simulink model "Project_adp_posmeas2_ver2"  (Simulink 7.3)
settings: Solver=ode45  StartTime=0.0  StopTime=25  RelTol=1e-3
libraries: dspmtrx3 x6, simulink x4
settings Model: Creator=GILL  LastModifiedBy=GILL

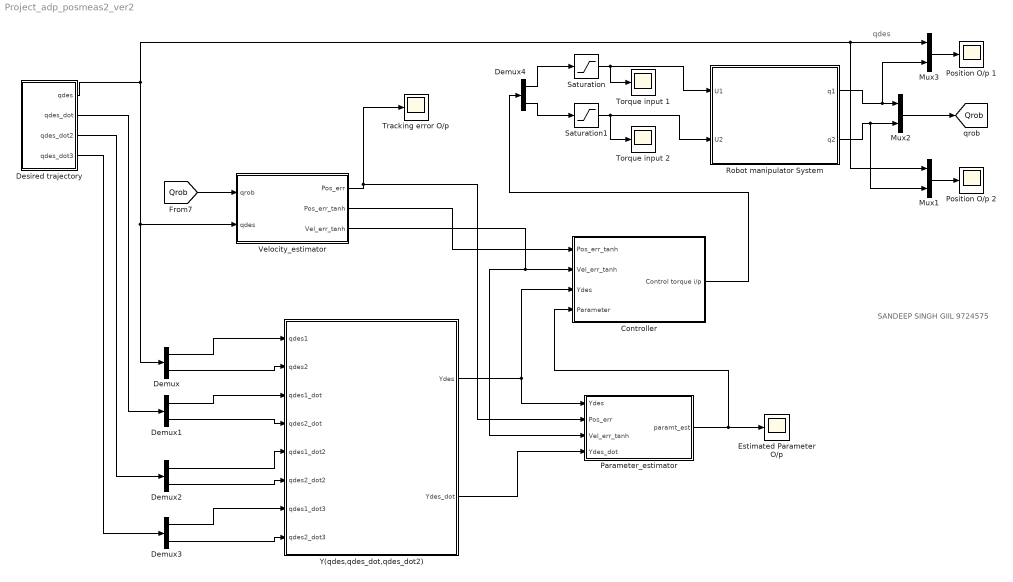
== system Project_adp_posmeas2_ver2 ==
  note: qdes
  note: SANDEEP SINGH GIIL
      | 9724575
  Controller : Subsystem
  Demux{,1..4} (5 alike) : Demux  Outputs=2
  Desired trajectory : Subsystem
  Estimated Parameter O/p : Scope
      settings: TimeRange=10  YMin=-4  SaveName=ScopeData3
  Mux1 : Mux  Inputs=2
  Mux2 : Mux  Inputs=2
  Mux3 : Mux  Inputs=2
  Parameter_estimator : Subsystem
  "Position O/p 1 " : Scope
      settings: TimeRange=8  YMin=-1.6  YMax=0.3999999999999999
  Position O/p 2 : Scope
      settings: TimeRange=10  YMin=-4  SaveName=ScopeData2
  Robot manipulator System : Subsystem
  Saturation : Saturate  UpperLimit=150  LowerLimit=-150
  Saturation1 : Saturate  UpperLimit=35  LowerLimit=-35
  Torque input 1 : Scope
      settings: TimeRange=10  YMin=-4  SaveName=ScopeData5
  Torque input 2 : Scope
      settings: TimeRange=10  YMin=-4  SaveName=ScopeData4
  Tracking error O/p : Scope
      settings: TimeRange=10  YMin=-4  SaveName=ScopeData7
  Velocity_estimator : Subsystem
  Y(qdes,qdes_dot,qdes_dot2) : Stateflow chart  TreatAsAtomicUnit=on
  tag scope: Qrob=global
  wires:
  Mux2/1 -> [Qrob]
  Robot manipulator System/1(q1) -> Mux2/1, Mux3/2
  Robot manipulator System/2(q2) -> Mux2/2, Mux1/2
  Mux3/1 -> "Position O/p 1 "/1
  [Qrob] -> Velocity_estimator/1(qrob)
  Desired trajectory/2(qdes_dot) -> Demux1/1
  Desired trajectory/3(qdes_dot2) -> Demux2/1
  Demux/2 -> Y(qdes,qdes_dot,qdes_dot2)/2(qdes2)
  Demux3/1 -> Y(qdes,qdes_dot,qdes_dot2)/7(qdes1_dot3)
  Demux3/2 -> Y(qdes,qdes_dot,qdes_dot2)/8(qdes2_dot3)
  Demux2/2 -> Y(qdes,qdes_dot,qdes_dot2)/6(qdes2_dot2)
  Demux2/1 -> Y(qdes,qdes_dot,qdes_dot2)/5(qdes1_dot2)
  Demux1/2 -> Y(qdes,qdes_dot,qdes_dot2)/4(qdes2_dot)
  Demux1/1 -> Y(qdes,qdes_dot,qdes_dot2)/3(qdes1_dot)
  Demux/1 -> Y(qdes,qdes_dot,qdes_dot2)/1(qdes1)
  Desired trajectory/4(qdes_dot3) -> Demux3/1
  Desired trajectory/1(qdes) -> Mux3/1, Mux1/1, Demux/1, Velocity_estimator/2(qdes)
  Velocity_estimator/1(Pos_err) -> Tracking error O/p/1, Parameter_estimator/2(Pos_err)
  Saturation/1 -> Torque input 1/1, Robot manipulator System/1(U1)
  Saturation1/1 -> Torque input 2/1, Robot manipulator System/2(U2)
  Demux4/2 -> Saturation1/1
  Demux4/1 -> Saturation/1
  Y(qdes,qdes_dot,qdes_dot2)/1(Ydes) -> Controller/3(Ydes), Parameter_estimator/1(Ydes)
  Controller/1(Control torque i/p) -> Demux4/1
  Velocity_estimator/2(Pos_err_tanh) -> Controller/1(Pos_err_tanh)
  Velocity_estimator/3(Vel_err_tanh) -> Controller/2(Vel_err_tanh), Parameter_estimator/3(Vel_err_tanh)
  Parameter_estimator/1(paramt_est) -> Estimated Parameter O/p/1, Controller/4(Parameter)
  Y(qdes,qdes_dot,qdes_dot2)/2(Ydes_dot) -> Parameter_estimator/4(Ydes_dot)
  Mux1/1 -> Position O/p 2/1

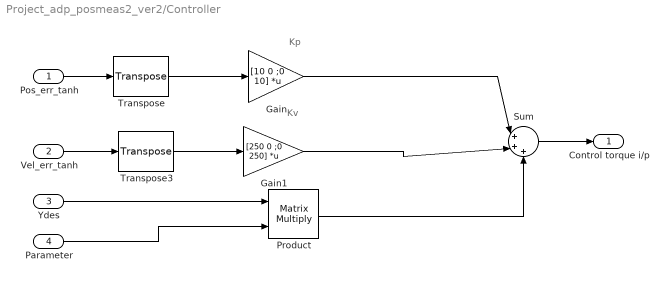
== system Project_adp_posmeas2_ver2/Controller ==
  note: Kp
  note: Kv
  Pos_err_tanh : Inport
  Vel_err_tanh : Inport  Port=2
  Ydes : Inport  Port=3
  Parameter : Inport  Port=4
  Gain : Gain  Gain=[10 0 ;0 10]  Multiplication=Matrix(K*u) (u vector)
  Gain1 : Gain  Gain=[250 0 ;0 250]  Multiplication=Matrix(K*u) (u vector)
  Product : Product  Multiplication=Matrix(*)  RndMeth=Zero
  Sum : Sum  Inputs=|+++
  Transpose : dspmtrx3/Transpose  SystemSampleTime=-1  Hermitian=off  overflowFlag=off
  Transpose3 : dspmtrx3/Transpose  SystemSampleTime=-1  Hermitian=off  overflowFlag=off
  Control torque i/p : Outport
  wires:
  Pos_err_tanh/1 -> Transpose/1
  Vel_err_tanh/1 -> Transpose3/1
  Product/1 -> Sum/3
  Gain/1 -> Sum/1
  Gain1/1 -> Sum/2
  Transpose/1 -> Gain/1
  Transpose3/1 -> Gain1/1
  Ydes/1 -> Product/1
  Parameter/1 -> Product/2
  Sum/1 -> Control torque i/p/1

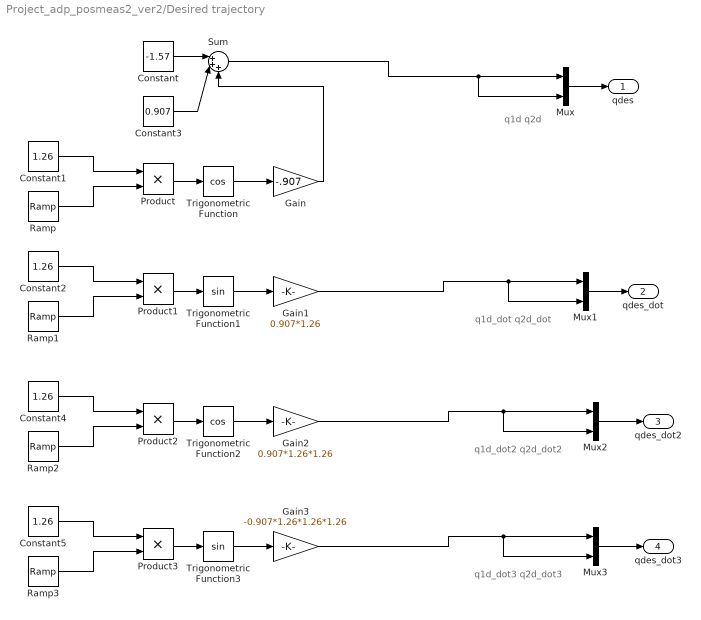
== system Project_adp_posmeas2_ver2/Desired trajectory ==
  note: q1d_dot
      | q2d_dot
  note: q1d
      | q2d
  note: q1d_dot2
      | q2d_dot2
  note: q1d_dot3
      | q2d_dot3
  Constant : Constant  Value=-1.57
  Constant{1..2,4..5} (4 alike) : Constant  Value=1.26
  Constant3 : Constant  Value=0.907
  Gain : Gain  Gain=-.907
  Gain1 : Gain  Gain=0.907*1.26
  Gain2 : Gain  Gain=0.907*1.26*1.26
  Gain3 : Gain  Gain=-0.907*1.26*1.26*1.26
  Mux{,1..3} (4 alike) : Mux  Inputs=2
  Product{,1..3} (4 alike) : Product  RndMeth=Zero
  Ramp{,1..3} (4 alike) : simulink/Sources/Ramp  SystemSampleTime=-1  slope=1  start=0  X0=0
  Sum : Sum  Inputs=|+++
  Trigonometric Function : Trigonometry  Operator=cos
  Trigonometric Function1 : Trigonometry
  Trigonometric Function2 : Trigonometry  Operator=cos
  Trigonometric Function3 : Trigonometry
  qdes : Outport
  qdes_dot : Outport  Port=2
  qdes_dot2 : Outport  Port=3
  qdes_dot3 : Outport  Port=4
  wires:
  Constant/1 -> Sum/1
  Constant1/1 -> Product/1
  Constant3/1 -> Sum/2
  Ramp/1 -> Product/2
  Product/1 -> Trigonometric Function/1
  Trigonometric Function/1 -> Gain/1
  Gain/1 -> Sum/3
  Constant2/1 -> Product1/1
  Ramp1/1 -> Product1/2
  Product1/1 -> Trigonometric Function1/1
  Trigonometric Function1/1 -> Gain1/1
  Constant4/1 -> Product2/1
  Ramp2/1 -> Product2/2
  Product2/1 -> Trigonometric Function2/1
  Trigonometric Function2/1 -> Gain2/1
  Mux/1 -> qdes/1
  Mux1/1 -> qdes_dot/1
  Mux2/1 -> qdes_dot2/1
  Gain2/1 -> Mux2/1, Mux2/2
  Gain1/1 -> Mux1/1, Mux1/2
  Sum/1 -> Mux/1, Mux/2
  Constant5/1 -> Product3/1
  Ramp3/1 -> Product3/2
  Product3/1 -> Trigonometric Function3/1
  Trigonometric Function3/1 -> Gain3/1
  Mux3/1 -> qdes_dot3/1
  Gain3/1 -> Mux3/1, Mux3/2

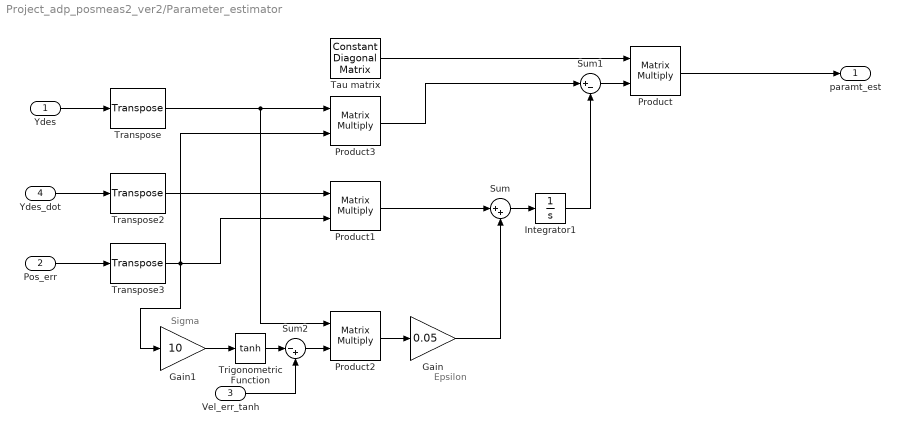
== system Project_adp_posmeas2_ver2/Parameter_estimator ==
  note: Epsilon
  note: Sigma
  Ydes : Inport
  Pos_err : Inport  Port=2
  Vel_err_tanh : Inport  Port=3
  Ydes_dot : Inport  Port=4
  Gain : Gain  Gain=0.05
  Gain1 : Gain  Gain=10
  Integrator1 : Integrator
  Product{,1..3} (4 alike) : Product  Multiplication=Matrix(*)  RndMeth=Zero
  Sum : Sum  Inputs=|++
  Sum1 : Sum  Inputs=|+-
  Sum2 : Sum  Inputs=|-+
  Tau matrix : dspmtrx3/Constant Diagonal Matrix  SystemSampleTime=-1  q=[1.6,2.5,8,10,2.5]  frame=off  dataType=Inherit from 'Constant(s) along diagonal'  isSigned=on  wordLen=16  udDataType=sfix(16)  fracBitsMode=Best precision  numFracBits=15
  Transpose : dspmtrx3/Transpose  SystemSampleTime=-1  Hermitian=off  overflowFlag=off
  Transpose2 : dspmtrx3/Transpose  SystemSampleTime=-1  Hermitian=off  overflowFlag=off
  Transpose3 : dspmtrx3/Transpose  SystemSampleTime=-1  Hermitian=off  overflowFlag=off
  Trigonometric Function : Trigonometry  Operator=tanh
  paramt_est : Outport
  wires:
  Ydes/1 -> Transpose/1
  Ydes_dot/1 -> Transpose2/1
  Transpose2/1 -> Product1/1
  Pos_err/1 -> Transpose3/1
  Transpose3/1 -> Product1/2, Gain1/1, Product3/2
  Gain1/1 -> Trigonometric Function/1
  Transpose/1 -> Product2/1, Product3/1
  Product2/1 -> Gain/1
  Product1/1 -> Sum/1
  Gain/1 -> Sum/2
  Sum/1 -> Integrator1/1
  Integrator1/1 -> Sum1/2
  Sum1/1 -> Product/2
  Tau matrix/1 -> Product/1
  Product/1 -> paramt_est/1
  Product3/1 -> Sum1/1
  Trigonometric Function/1 -> Sum2/1
  Sum2/1 -> Product2/2
  Vel_err_tanh/1 -> Sum2/2

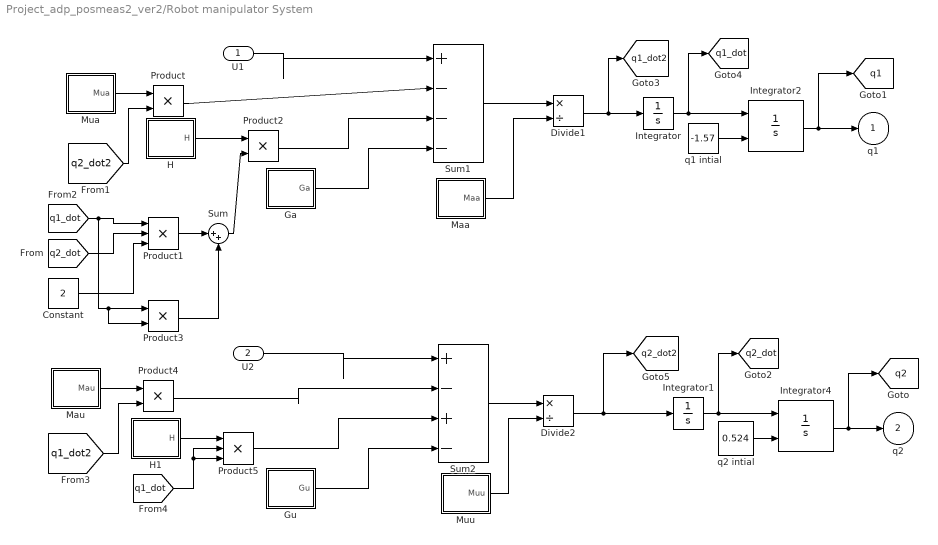
== system Project_adp_posmeas2_ver2/Robot manipulator System ==
  U1 : Inport
  U2 : Inport  Port=2
  Constant : Constant  Value=2
  Divide1 : Product  Inputs=*/
  Divide2 : Product  Inputs=*/
  Ga : Subsystem
  Gu : Subsystem
  H : Subsystem
  H1 : Subsystem
  Integrator : Integrator
  Integrator1 : Integrator
  Integrator2 : Integrator  InitialConditionSource=external
  Integrator4 : Integrator  InitialConditionSource=external
  Maa : Subsystem
  Mau : Subsystem
  Mua : Subsystem
  Muu : Subsystem
  Product{,2..4} (4 alike) : Product  RndMeth=Zero
  Product1 : Product  Inputs=3  RndMeth=Zero
  Product5 : Product  Inputs=3  RndMeth=Zero
  Sum : Sum  Inputs=|++
  Sum1 : Sum  Inputs=|+---
  Sum2 : Sum  Inputs=|+-+-
  "q1 intial " : Constant  Value=-1.57
  "q2 intial " : Constant  Value=0.524
  q1 : Outport
  q2 : Outport  Port=2
  tag scope: q1=global, q1_dot2=global, q1_dot=global, q2=global, q2_dot2=global, q2_dot=global
  wires:
  Mua/1(Mua) -> Product/1
  [q2_dot2] -> Product/2
  Product/1 -> Sum1/2
  U1/1 -> Sum1/1
  [q1_dot] -> Product1/1, Product3/1, Product3/2
  [q2_dot] -> Product1/2
  Constant/1 -> Product1/3
  H/1(H) -> Product2/1
  Product1/1 -> Sum/1
  Sum/1 -> Product2/2
  Product2/1 -> Sum1/3
  Product3/1 -> Sum/2
  Ga/1(Ga) -> Sum1/4
  Sum1/1 -> Divide1/1
  Maa/1(Maa) -> Divide1/2
  Divide1/1 -> Integrator/1, [q1_dot2]
  Integrator/1 -> Integrator2/1, [q1_dot]
  "q1 intial "/1 -> Integrator2/2
  Integrator2/1 -> q1/1, [q1]
  U2/1 -> Sum2/1
  Sum2/1 -> Divide2/1
  Muu/1(Muu) -> Divide2/2
  Mau/1(Mau) -> Product4/1
  [q1_dot2] -> Product4/2
  Product4/1 -> Sum2/2
  H1/1(H) -> Product5/1
  [q1_dot] -> Product5/2, Product5/3
  Product5/1 -> Sum2/3
  Gu/1(Gu) -> Sum2/4
  Divide2/1 -> Integrator1/1, [q2_dot2]
  Integrator1/1 -> Integrator4/1, [q2_dot]
  "q2 intial "/1 -> Integrator4/2
  Integrator4/1 -> q2/1, [q2]

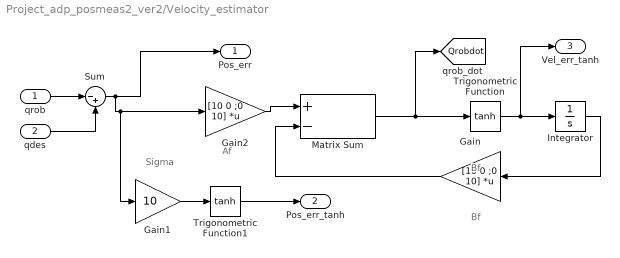
== system Project_adp_posmeas2_ver2/Velocity_estimator ==
  note: Bf
  note: Af
  note: Sigma
  note: Bf
  qrob : Inport
  qdes : Inport  Port=2
  Gain : Gain  Gain=[10 0 ;0 10]  Multiplication=Matrix(K*u) (u vector)
  Gain1 : Gain  Gain=10
  Gain2 : Gain  Gain=[10 0 ;0 10]  Multiplication=Matrix(K*u) (u vector)
  Integrator : Integrator
  Matrix Sum : Sum  Inputs=+-
  Sum : Sum  Inputs=|-+
  Trigonometric Function : Trigonometry  Operator=tanh
  Trigonometric Function1 : Trigonometry  Operator=tanh
  Pos_err : Outport
  Pos_err_tanh : Outport  Port=2
  Vel_err_tanh : Outport  Port=3
  tag scope: Qrobdot=global
  wires:
  qrob/1 -> Sum/1
  qdes/1 -> Sum/2
  Sum/1 -> Pos_err/1, Gain2/1, Gain1/1
  Gain2/1 -> Matrix Sum/1
  Trigonometric Function/1 -> Integrator/1, Vel_err_tanh/1
  Gain/1 -> Matrix Sum/2
  Integrator/1 -> Gain/1
  Matrix Sum/1 -> Trigonometric Function/1, [Qrobdot]
  Gain1/1 -> Trigonometric Function1/1
  Trigonometric Function1/1 -> Pos_err_tanh/1

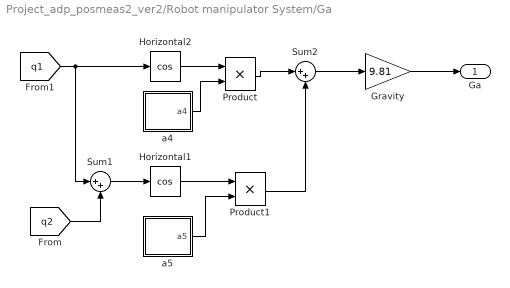
== system Project_adp_posmeas2_ver2/Robot manipulator System/Ga ==
  Gravity : Gain  Gain=9.81
  Horizontal1 : Trigonometry  Operator=cos
  Horizontal2 : Trigonometry  Operator=cos
  Product : Product  RndMeth=Zero
  Product1 : Product  RndMeth=Zero
  Sum1 : Sum  Inputs=|++
  Sum2 : Sum  Inputs=|++
  a4 : Subsystem
  a5 : Subsystem
  Ga : Outport
  wires:
  [q1] -> Horizontal2/1, Sum1/1
  Sum1/1 -> Horizontal1/1
  Horizontal2/1 -> Product/1
  a4/1(a4) -> Product/2
  Product/1 -> Sum2/1
  Sum2/1 -> Gravity/1
  Gravity/1 -> Ga/1
  Horizontal1/1 -> Product1/1
  a5/1(a5) -> Product1/2
  Product1/1 -> Sum2/2
  [q2] -> Sum1/2

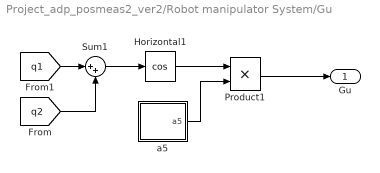
== system Project_adp_posmeas2_ver2/Robot manipulator System/Gu ==
  Horizontal1 : Trigonometry  Operator=cos
  Product1 : Product  RndMeth=Zero
  Sum1 : Sum  Inputs=|++
  a5 : Subsystem
  Gu : Outport
  wires:
  [q1] -> Sum1/1
  Sum1/1 -> Horizontal1/1
  [q2] -> Sum1/2
  Horizontal1/1 -> Product1/1
  a5/1(a5) -> Product1/2
  Product1/1 -> Gu/1

== system Project_adp_posmeas2_ver2/Robot manipulator System/H ==
  Constant : Constant  Value=-1
  Horizontal2 : Trigonometry
  Product : Product  Inputs=3  RndMeth=Zero
  a2 : Subsystem
  H : Outport
  wires:
  Horizontal2/1 -> Product/1
  a2/1(a2) -> Product/2
  Constant/1 -> Product/3
  Product/1 -> H/1
  [q2] -> Horizontal2/1

== system Project_adp_posmeas2_ver2/Robot manipulator System/H1 ==
  Constant : Constant  Value=-1
  Horizontal2 : Trigonometry
  Product : Product  Inputs=3  RndMeth=Zero
  a2 : Subsystem
  H : Outport
  wires:
  Horizontal2/1 -> Product/1
  a2/1(a2) -> Product/2
  Constant/1 -> Product/3
  Product/1 -> H/1
  [q2] -> Horizontal2/1

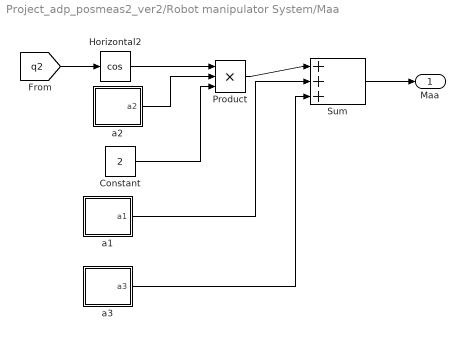
== system Project_adp_posmeas2_ver2/Robot manipulator System/Maa ==
  Constant : Constant  Value=2
  Horizontal2 : Trigonometry  Operator=cos
  Product : Product  Inputs=3  RndMeth=Zero
  Sum : Sum  Inputs=|+++
  a1 : Subsystem
  a2 : Subsystem
  a3 : Subsystem
  Maa : Outport
  wires:
  Horizontal2/1 -> Product/1
  a2/1(a2) -> Product/2
  Constant/1 -> Product/3
  Product/1 -> Sum/1
  a1/1(a1) -> Sum/2
  a3/1(a3) -> Sum/3
  Sum/1 -> Maa/1
  [q2] -> Horizontal2/1

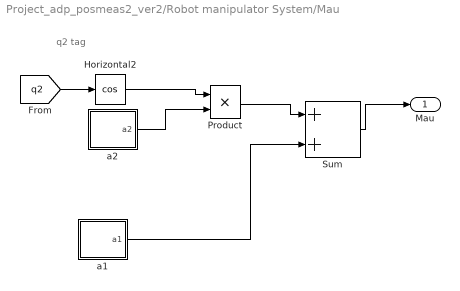
== system Project_adp_posmeas2_ver2/Robot manipulator System/Mau ==
  note: q2
      | tag
  Horizontal2 : Trigonometry  Operator=cos
  Product : Product  RndMeth=Zero
  Sum : Sum  Inputs=|++
  a1 : Subsystem
  a2 : Subsystem
  Mau : Outport
  wires:
  Horizontal2/1 -> Product/1
  a2/1(a2) -> Product/2
  Product/1 -> Sum/1
  a1/1(a1) -> Sum/2
  Sum/1 -> Mau/1
  [q2] -> Horizontal2/1

== system Project_adp_posmeas2_ver2/Robot manipulator System/Mua ==
  Horizontal2 : Trigonometry  Operator=cos
  Product : Product  RndMeth=Zero
  Sum : Sum  Inputs=|++
  a1 : Subsystem
  a2 : Subsystem
  Mua : Outport
  wires:
  Horizontal2/1 -> Product/1
  a2/1(a2) -> Product/2
  Product/1 -> Sum/1
  a1/1(a1) -> Sum/2
  Sum/1 -> Mua/1
  [q2] -> Horizontal2/1

== system Project_adp_posmeas2_ver2/Robot manipulator System/Muu ==
  I2 : Constant  Value=5/12
  Lc2 : Constant  Value=0.5
  M2 : Constant  Value=5
  Product12 : Product  Inputs=3  RndMeth=Zero
  Sum10 : Sum  Inputs=|++
  Muu : Outport
  wires:
  M2/1 -> Product12/1
  Lc2/1 -> Product12/2, Product12/3
  I2/1 -> Sum10/1
  Product12/1 -> Sum10/2
  Sum10/1 -> Muu/1

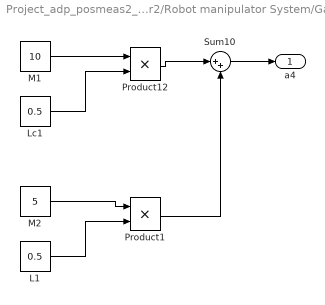
== system Project_adp_posmeas2_ver2/Robot manipulator System/Ga/a4 ==
  L1 : Constant  Value=0.5
  Lc1 : Constant  Value=0.5
  M1 : Constant  Value=10
  M2 : Constant  Value=5
  Product1 : Product  RndMeth=Zero
  Product12 : Product  RndMeth=Zero
  Sum10 : Sum  Inputs=|++
  a4 : Outport
  wires:
  M1/1 -> Product12/1
  Lc1/1 -> Product12/2
  Sum10/1 -> a4/1
  M2/1 -> Product1/1
  L1/1 -> Product1/2
  Product1/1 -> Sum10/2
  Product12/1 -> Sum10/1

== system Project_adp_posmeas2_ver2/Robot manipulator System/Ga/a5 ==
  Lc2 : Constant  Value=0.5
  M2 : Constant  Value=5
  Product12 : Product  RndMeth=Zero
  a5 : Outport
  wires:
  M2/1 -> Product12/1
  Lc2/1 -> Product12/2
  Product12/1 -> a5/1

== system Project_adp_posmeas2_ver2/Robot manipulator System/Gu/a5 ==
  Lc2 : Constant  Value=0.5
  M2 : Constant  Value=5
  Product12 : Product  RndMeth=Zero
  a5 : Outport
  wires:
  M2/1 -> Product12/1
  Lc2/1 -> Product12/2
  Product12/1 -> a5/1

== system Project_adp_posmeas2_ver2/Robot manipulator System/H/a2 ==
  L1 : Constant
  Lc2 : Constant  Value=0.5
  M2 : Constant  Value=5
  Product12 : Product  Inputs=3  RndMeth=Zero
  a2 : Outport
  wires:
  M2/1 -> Product12/1
  Lc2/1 -> Product12/2
  L1/1 -> Product12/3
  Product12/1 -> a2/1

== system Project_adp_posmeas2_ver2/Robot manipulator System/H1/a2 ==
  L1 : Constant
  Lc2 : Constant  Value=0.5
  M2 : Constant  Value=5
  Product12 : Product  Inputs=3  RndMeth=Zero
  a2 : Outport
  wires:
  M2/1 -> Product12/1
  Lc2/1 -> Product12/2
  L1/1 -> Product12/3
  Product12/1 -> a2/1

== system Project_adp_posmeas2_ver2/Robot manipulator System/Maa/a1 ==
  I2 : Constant  Value=5/12
  Lc2 : Constant  Value=0.5
  M2 : Constant  Value=5
  Product12 : Product  Inputs=3  RndMeth=Zero
  Sum10 : Sum  Inputs=|++
  a1 : Outport
  wires:
  M2/1 -> Product12/1
  Lc2/1 -> Product12/2, Product12/3
  I2/1 -> Sum10/1
  Product12/1 -> Sum10/2
  Sum10/1 -> a1/1

== system Project_adp_posmeas2_ver2/Robot manipulator System/Maa/a2 ==
  L1 : Constant
  Lc2 : Constant  Value=0.5
  M2 : Constant  Value=5
  Product12 : Product  Inputs=3  RndMeth=Zero
  a2 : Outport
  wires:
  M2/1 -> Product12/1
  Lc2/1 -> Product12/2
  L1/1 -> Product12/3
  Product12/1 -> a2/1

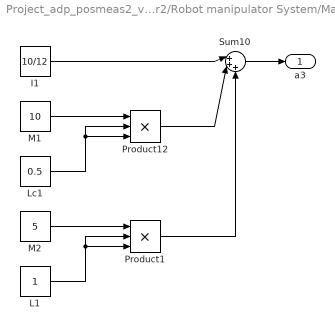
== system Project_adp_posmeas2_ver2/Robot manipulator System/Maa/a3 ==
  I1 : Constant  Value=10/12
  L1 : Constant
  Lc1 : Constant  Value=0.5
  M1 : Constant  Value=10
  M2 : Constant  Value=5
  Product1 : Product  Inputs=3  RndMeth=Zero
  Product12 : Product  Inputs=3  RndMeth=Zero
  Sum10 : Sum  Inputs=|+++
  a3 : Outport
  wires:
  M1/1 -> Product12/1
  Lc1/1 -> Product12/2, Product12/3
  I1/1 -> Sum10/1
  Product12/1 -> Sum10/2
  Sum10/1 -> a3/1
  M2/1 -> Product1/1
  L1/1 -> Product1/2, Product1/3
  Product1/1 -> Sum10/3

== system Project_adp_posmeas2_ver2/Robot manipulator System/Mau/a1 ==
  I2 : Constant  Value=5/12
  Lc2 : Constant  Value=0.5
  M2 : Constant  Value=5
  Product12 : Product  Inputs=3  RndMeth=Zero
  Sum10 : Sum  Inputs=|++
  a1 : Outport
  wires:
  M2/1 -> Product12/1
  Lc2/1 -> Product12/2, Product12/3
  I2/1 -> Sum10/1
  Product12/1 -> Sum10/2
  Sum10/1 -> a1/1

== system Project_adp_posmeas2_ver2/Robot manipulator System/Mau/a2 ==
  L1 : Constant
  Lc2 : Constant  Value=0.5
  M2 : Constant  Value=5
  Product12 : Product  Inputs=3  RndMeth=Zero
  a2 : Outport
  wires:
  M2/1 -> Product12/1
  Lc2/1 -> Product12/2
  L1/1 -> Product12/3
  Product12/1 -> a2/1

== system Project_adp_posmeas2_ver2/Robot manipulator System/Mua/a1 ==
  I2 : Constant  Value=5/12
  Lc2 : Constant  Value=0.5
  M2 : Constant  Value=5
  Product12 : Product  Inputs=3  RndMeth=Zero
  Sum10 : Sum  Inputs=|++
  a1 : Outport
  wires:
  M2/1 -> Product12/1
  Lc2/1 -> Product12/2, Product12/3
  I2/1 -> Sum10/1
  Product12/1 -> Sum10/2
  Sum10/1 -> a1/1

== system Project_adp_posmeas2_ver2/Robot manipulator System/Mua/a2 ==
  L1 : Constant
  Lc2 : Constant  Value=0.5
  M2 : Constant  Value=5
  Product12 : Product  Inputs=3  RndMeth=Zero
  a2 : Outport
  wires:
  M2/1 -> Product12/1
  Lc2/1 -> Product12/2
  L1/1 -> Product12/3
  Product12/1 -> a2/1

== matlab function Y(qdes,qdes_dot,qdes_dot2) ==
  data: qdes1 input double; Ydes output double; qdes2 input double; qdes1_dot input double; qdes2_dot input double; qdes1_dot2 input double; qdes2_dot2 input double; qdes1_dot3 input double; qdes2_dot3 input double; Ydes_dot output double
function [Ydes,Ydes_dot]  = fcn(qdes1,qdes2,qdes1_dot,qdes2_dot,qdes1_dot2,qdes2_dot2,qdes1_dot3,qdes2_dot3)
%#eml

a11 = qdes1_dot2 + qdes2_dot2;
a12 = (cos(qdes2)*(2*qdes1_dot2+qdes2_dot2)) - (sin(qdes2)*(2*qdes1_dot*qdes2_dot));
a13 = qdes1_dot2;
a14 = 9.8 * cos(qdes1);
a15 = 9.8 * cos(qdes1 + qdes2);
a21 = qdes1_dot2 + qdes2_dot2;
a22 = (qdes1_dot2*cos(qdes2))+(qdes1_dot*qdes1_dot* sin(qdes2));
a23 = 0; 
a24 = 0;
a25 = cos(qdes1 + qdes2);
Ydes = [a11,a12,a13,a14,a15;a21,a22,a23,a24,a25];

b11 = qdes1_dot3 + qdes2_dot3;
b12 = (cos(qdes2)*((2*qdes1_dot3)+qdes2_dot3-(qdes1_dot*qdes1_dot)-(2*qdes1_dot*qdes2_dot)))-(sin(qdes2)*((2*qdes1_dot2)+qdes2_dot2+(2*qdes1_dot)+(2*qdes1_dot*qdes2_dot2)+(2*qdes1_dot2*qdes2_dot)));
b13 = qdes1_dot3;
b14 = -9.8*sin(qdes1);
b15 = -2*9.8* sin(qdes1 + qdes2);
b21 = qdes1_dot3 + qdes2_dot3;
b22 = (sin(qdes2)*(2*qdes1_dot-qdes1_dot2)) + (cos(qdes2)*(qdes1_dot3+(qdes1_dot*qdes1_dot)));
b23 = 0;
b24 = 0;
b25 = -2*sin(qdes1 + qdes2);
Ydes_dot = [b11,b12,b13,b14,b15;b21,b22,b23,b24,b25];
